simulink model "Longitudinaldynamicmodel_SmartFortwo"  (R2021b)
settings: Solver=FixedStepAuto  StartTime=0.0  StopTime=1  FixedStep=0.01  RelTol=1e-3
undefined symbols (not defined in the file): DiscIntNeverNeededParam, VehMass
libraries: Constant_Environment x1, Driver_PI x1, Longitudinal_DrivingCycles x1, Acceleration_Calculation x1, Air_Resistance x1, Roll_Resistance x1, Slope_Resistance x1, Constant_Power_Source x1, Simple_Auxiliary x1, Electric_Drive_Tabled_Consumption x1, Gear_Stage x1, DCAC_Converter x1
(part 2 of 3)

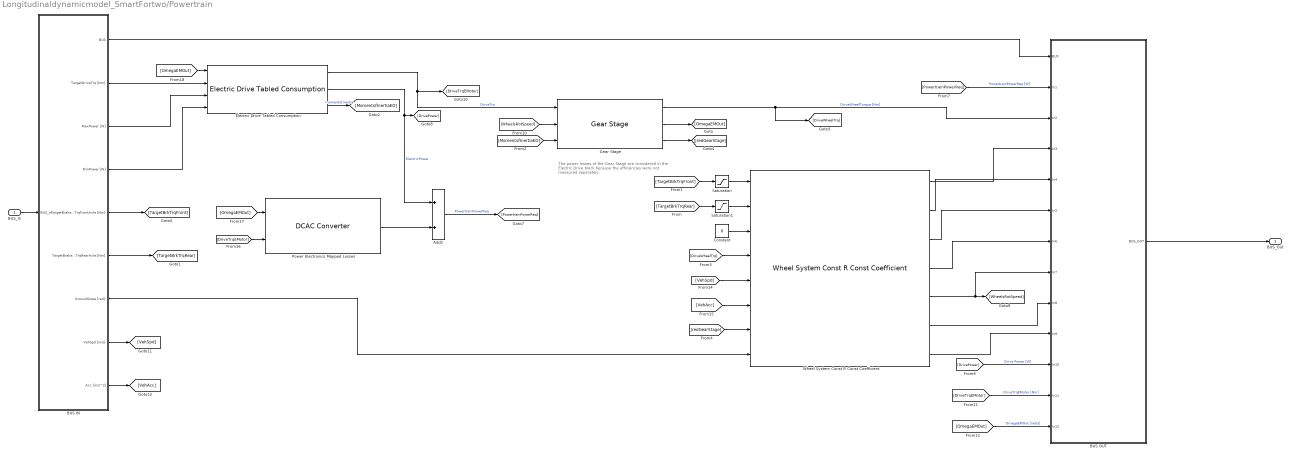
== system Longitudinaldynamicmodel_SmartFortwo/Powertrain ==
  note: The power losses of the Gear Stage are considered
      | in the Electric Drive block because the efficiencies were
      | not measured separately.
  BUS_In : Inport
  Add2 : Sum
  BUS IN : Subsystem
      mask help:
      | <Author> Alexander Koch based on Stefan Müller, Stephan Rohr
      | <Date> 02/05/2017
      |
      | <Description>
      | Automated BUS IN Block for the Bus System. After the Bus In is connected and receives signals it is possible to choose the required signals by clicking on the block. After choosing the signals it is possible to push the Refresh button. This button builds the required amount of outputs, connects the Bus Selector and the Outputs and rename all the outputs with the corresponding signal name.
      |
      | The Block automaticlly disconnects the link to the library block after opening the first time
      |
      | <Parameters>
      | -
      |
      | <Inputs>
      | Bus [Bus]
      |
      | <Outputs>
      | Bus [Bus]
      | SignalName[-]
      mask init:
      | BusInInitFct()
      settings: OpenFcn=|
      | set_param(gcb(),'LinkStatus','none')
      | open_system(gcb(),'mask')
      | open_system(strcat(gcb(),'/Bus Selector'),'Parameter')
      mask DialogControl ParameterGroupVar Prompt: Refresh
      mask DialogControl RefreshOutputs Prompt: Refresh all Output Names
      mask DialogControl RefreshOutputs Callback: BusInInitFct()
  BUS OUT : Subsystem  mask{NumberofInputs=12, NameSys='Powertrain'}
      mask prompts: NumberofInputs "Numper of costum inputs"; NameSys "Name of Bus Subsystem"
      mask help:
      | <Author> Alexander Koch based on Stefan Müller, Stephan Rohr
      | <Date> 02/05/2017
      |
      | <Description>
      | Automated BUS Out Block for the Bus System. Allows to enter the Number of costum inputs and the name of the bus system. After entering the parameters the required amout of Inputs are built and connected to the Bus Creator. The signal names that are connected to the inputs In1, ..., InN are automatically adopted at the Bus signal names and can be found in the Bus under the name of the Bus Subsystem. If the signal (line) to the Inport has no name, the name of the previous blocks outport is taken. If this is not possible, the name if the previous block is taken for the Bus signal name.
      |
      | Additional, there are two buttons. The Refresh Input Names refreshes all Input Names. This is required if signal names are changed or signals are connected for the first time. To build a new system or if another Subsystem is added between existing subsystems, the Refresh Bus Selector is required at every subsystem that is calculated after the new subsystem.
      |
      | The Block automaticlly disconnects the link to the library block after opening the first time
      |
      | <Parameters>
      | Number of costum inputs [-]
      | Name of Bus Subsystem ['abc']
      |
      | <Inputs>
      | Bus [Bus]
      | In1 [ ]
      |
      | <Outputs>
      | Bus [Bus]
      mask init:
      | BusRefreshInputs()
      settings: OpenFcn=|
      | set_param(gcb(),'LinkStatus','none')
      | open_system(gcb(),'mask')
      mask DialogControl Container3 Prompt: Refresh
      mask DialogControl RefreshInputNames Prompt: Refresh Input Names
      mask DialogControl RefreshInputNames Callback: BusRefreshLineNames()
      mask DialogControl RefreshBusSelector Prompt: Refresh Bus Selector
      mask DialogControl RefreshBusSelector Callback: BusRefreshBusSelector()
  Constant : Constant  Value=0
  Electric Drive Tabled Consumption : Electric_Drive_Tabled_Consumption/Electric Drive Tabled Consumption  inertia=0.03  mass=1  OM_M_Pel_Map=[-4936.58960230285,-4918.30593710914,-4900.02227191542,-4881.73860672171,-4863.45494152799,-4845.17127633428,-4826.88761114056,-4808.60394594685,-4790.32028075314,-4772.03661555942,-4753.75295036571,-4735.46928517199,-4717.18561997828,-4698.90195478456,-4680.61828959085,-4662.33462439714,-5185.11366506308,-5115.90505550168,-4971.88831379428,-4292.42207149109,-4491.53844424213,-4496.68242435772,-3427.33324656741,-3576.85553346338,-4862.92900152083,-6633.71124555647,-8634.89642494398,-4640.86226177616,-3090.77270566202,-3263.80065362687,-3496.71961565219,-3476.52721907770,-3156.42090156138,-3528.67393415159,-3943.07312633913,-1726.22025060580,0,-284.730200184838,-3008.08986597435,-2771.67771496470,-1854.05476499352,-1637.18751237163,-1896.50054154000,-1755.41745851923,-1704.42214651483,-1837.80488310502,-2503.90899285254,-3057.39048489453,-3952.42911160673,-4269.34747269463,-4242.89467363708,-4204.95309118347,-4162.48827607546,-4121.62290347057,-4107.04807601649,-4077.92876166182,-4033.68022948992,-4001.70150845442,-3928.04097239828,-3892.85157240146,-3860.86018153553,-3833.69713173239,-3822.33875240511,-3752.79975327265,-3710.92826749583,-3673.11813401635,-3650.11543119095,-3617.55425584301,-3571.83464080449,-3546.22881032664,-3521.91492991431,-3503.51647273559,-3486.02852972273,-3456.08511172243,-3426.20785526970,-3393.22836186158,-3347.26416827824,-3315.74459108047,-3296.14668080983,-3259.87537919135,-3239.41741836494,-3209.57517612393,-3171.72598576032,-3145.46589033245,-3114.73817397058,-3096.82260491367,-3083.69891203201,-3028.53546438293,-2988.91641709166,-2952.55258487163,-2929.27984242158,-2918.30740683215,-2873.01765728202,-2827.29316803929,-2793.78872353345,-2774.19345844693,-2759.15266733751,-2740.21288555482,-2712.48373689461,-2700.63324424749,-2672.00671871173,-2652.70867089400,-2641.22885174613,-2609.92742749761,-2590.43803114605,-2552.66583691581,-2523.45685997718,-2500.24253764220,-2459.00798676327,-2438.92186521623,-2407.06238415750,-2382.52048698444,-2363.76081048896,-2359.58944186339,-2345.68370297819,-2308.79818370909,-2284.46288528949,-2265.18882858931,-2236.12233498368,-2202.96158268492,-2190.88870254505,-2161.55169347863,-2130.75207473189,-2100.15228890542,-2083.00628884149,-2065.03289270050,-2037.48564486677,-2023.21148849436,-2003.60224940543,-1985.10896747608,-1973.43738121688,-1954.15563352281,-1936.49980013294,-1927.41778977736,-1881.51131814734,-1833.22793591959,-1812.31297236205,-1791.45842660955,-1776.91834015446,-1771.92258671922,-1753.46238532805,-1738.43989396041,-1734.97839912883,-1730.47565907493,-1707.15901890688,-1688.09192045326,-1670.78344209104,-1655.54467412356,-1639.03791207785,-1627.05930580792,-1604.77335708724,-1587.38076614672,-1561.52550139142,-1537.72571637804,-1510.39275514847,-1470.58244002962,-1453.15319676168,-1410.88893113516,-1321.00360833135,-1269.23703081773,-1254.49077239222,-1241.38468901509,-1229.32636706052,-1202.25203822531,-1184.94448226145,-1158.42848336410,-1136.20405147524,-1126.39720329839,-1106.37247296839,-1094.85258153359,-1077.77222327341,-1048.86179199116,-1029.92385889766,-1012.51433236396,-1002.83703023995,-999.671500372368,-987.625469219025,-971.502457237745,-944.816892286739,-933.727512080550,-927.465392779959,-908.500787820009,-892.918090905503,-877.260552760021,-857.206260698465,-846.212481472991,-838.179969253041,-830.641165096547,-807.984200911199,-798.124054496656,-792.518428146118,-765.637990495186,-746.212652936259,-712.453130410888,-696.980692898239,-691.969161426306,-672.764183049685,-663.434558579034,-643.975843820281,-631.350187559368,-617.856740921016,-610.270426732149,-591.410647728663,-578.788040954300,-569.720295539698,-556.273882509573,-549.087372350833,-540.864224298053,-525.831584341530,-513.205249528202,-497.309584323254,-484.661307411820,-466.385751839651,-461.707756868834,-448.056335365480,-434.987633724325,-427.031177729718,-408.480763130817,-385.296760841008,-359.496386063347,-344.092316830198,-331.596273553197,-323.279256624167 ...(+563781 chars)]  M_MotVector=[-135,-134.500000000000,-134,-133.500000000000,-133,-132.500000000000,-132,-131.500000000000,-131,-130.500000000000,-130,-129.500000000000,-129,-128.500000000000,-128,-127.500000000000,-127,-126.500000000000,-126,-125.500000000000,-125,-124.500000000000,-124,-123.500000000000,-123,-122.500000000000,-122,-121.500000000000,-121,-120.500000000000,-120,-119.500000000000,-119,-118.500000000000,-118,-117.500000000000,-117,-116.500000000000,-116,-115.500000000000,-115,-114.500000000000,-114,-113.500000000000,-113,-112.500000000000,-112,-111.500000000000,-111,-110.500000000000,-110,-109.500000000000,-109,-108.500000000000,-108,-107.500000000000,-107,-106.500000000000,-106,-105.500000000000,-105,-104.500000000000,-104,-103.500000000000,-103,-102.500000000000,-102,-101.500000000000,-101,-100.500000000000,-100,-99.5000000000000,-99,-98.5000000000000,-98,-97.5000000000000,-97,-96.5000000000000,-96,-95.5000000000000,-95,-94.5000000000000,-94,-93.5000000000000,-93,-92.5000000000000,-92,-91.5000000000000,-91,-90.5000000000000,-90,-89.5000000000000,-89,-88.5000000000000,-88,-87.5000000000000,-87,-86.5000000000000,-86,-85.5000000000000,-85,-84.5000000000000,-84,-83.5000000000000,-83,-82.5000000000000,-82,-81.5000000000000,-81,-80.5000000000000,-80,-79.5000000000000,-79,-78.5000000000000,-78,-77.5000000000000,-77,-76.5000000000000,-76,-75.5000000000000,-75,-74.5000000000000,-74,-73.5000000000000,-73,-72.5000000000000,-72,-71.5000000000000,-71,-70.5000000000000,-70,-69.5000000000000,-69,-68.5000000000000,-68,-67.5000000000000,-67,-66.5000000000000,-66,-65.5000000000000,-65,-64.5000000000000,-64,-63.5000000000000,-63,-62.5000000000000,-62,-61.5000000000000,-61,-60.5000000000000,-60,-59.5000000000000,-59,-58.5000000000000,-58,-57.5000000000000,-57,-56.5000000000000,-56,-55.5000000000000,-55,-54.5000000000000,-54,-53.5000000000000,-53,-52.5000000000000,-52,-51.5000000000000,-51,-50.5000000000000,-50,-49.5000000000000,-49,-48.5000000000000,-48,-47.5000000000000,-47,-46.5000000000000,-46,-45.5000000000000,-45,-44.5000000000000,-44,-43.5000000000000,-43,-42.5000000000000,-42,-41.5000000000000,-41,-40.5000000000000,-40,-39.5000000000000,-39,-38.5000000000000,-38,-37.5000000000000,-37,-36.5000000000000,-36,-35.5000000000000,-35,-34.5000000000000,-34,-33.5000000000000,-33,-32.5000000000000,-32,-31.5000000000000,-31,-30.5000000000000,-30,-29.5000000000000,-29,-28.5000000000000,-28,-27.5000000000000,-27,-26.5000000000000,-26,-25.5000000000000,-25,-24.5000000000000,-24,-23.5000000000000,-23,-22.5000000000000,-22,-21.5000000000000,-21,-20.5000000000000,-20,-19.5000000000000,-19,-18.5000000000000,-18,-17.5000000000000,-17,-16.5000000000000,-16,-15.5000000000000,-15,-14.5000000000000,-14,-13.5000000000000,-13,-12.5000000000000,-12,-11.5000000000000,-11,-10.5000000000000,-10,-9.50000000000000,-9,-8.50000000000000,-8,-7.50000000000000,-7,-6.50000000000000,-6,-5.50000000000000,-5,-4.50000000000000,-4,-3.50000000000000,-3,-2.50000000000000,-2,-1.50000000000000,-1,-0.500000000000000,0,0.500000000000000,1,1.50000000000000,2,2.50000000000000,3,3.50000000000000,4,4.50000000000000,5,5.50000000000000,6,6.50000000000000,7,7.50000000000000,8,8.50000000000000,9,9.50000000000000,10,10.5000000000000,11,11.5000000000000,12,12.5000000000000,13,13.5000000000000,14,14.5000000000000,15,15.5000000000000,16,16.5000000000000,17,17.5000000000000,18,18.5000000000000,19,19.5000000000000,20,20.5000000000000,21,21.5000000000000,22,22.5000000000000,23,23.5000000000000,24,24.5000000000000,25,25.5000000000000,26,26.5000000000000,27,27.5000000000000,28,28.5000000000000,29,29.5000000000000,30,30.5000000000000,31,31.5000000000000,32,32.5000000000000,33,33.5000000000000,34,34.5000000000000,35,35.5000000000000,36,36.5000000000000,37,37.5000000000000,38,38.5000000000000,39,39.5000000000000,40,40.5000000000000,41,41.5000000000000,42,42.5000000000000,43,43.5000000000000,44,44.5000000000000,45,45.5000000000000,46,46.5000000000000,47,47.5000000000000,48,48.5000000000000,49,49.5000000000000,50 ...(+1736 chars)]  OM_MotVector=[0,11.6256677293860,23.2513354587719,34.8770031881579,46.5026709175438,58.1283386469298,69.7540063763158,81.3796741057017,93.0053418350877,104.631009564474,116.256677293860,127.882345023246,139.508012752632,151.133680482017,162.759348211403,174.385015940789,186.010683670175,197.636351399561,209.262019128947,220.887686858333,232.513354587719,244.139022317105,255.764690046491,267.390357775877,279.016025505263,290.641693234649,302.267360964035,313.893028693421,325.518696422807,337.144364152193,348.770031881579,360.395699610965,372.021367340351,383.647035069737,395.272702799123,406.898370528509,418.524038257894,430.149705987280,441.775373716666,453.401041446052,465.026709175438,476.652376904824,488.278044634210,499.903712363596,511.529380092982,523.155047822368,534.780715551754,546.406383281140,558.032051010526,569.657718739912,581.283386469298,592.909054198684,604.534721928070,616.160389657456,627.786057386842,639.411725116228,651.037392845614,662.663060575000,674.288728304386,685.914396033772]  M_Full_Load=[128 128 128 127 127 126 126 126 126 124 119 114 109 103 100 94 89 85 79 75 70 68 67 65 63 62 60 58 59 60 62 63 63 62 61 60 58 57 55 53 51 50 48 46 45 43 42 40 39 38 36 35 34 32 31 30 29 28 26 25 24]  OM_Full_Load=[0 11.4144533080429 22.8289066160858 34.2433599241288 45.6578132321717 57.1769862953342 68.5914396033771 80.0058929114201 91.4203462194630 102.834799527506 114.249252835549 125.663706143592 137.078159451635 148.492612759678 160.011785822840 171.426239130883 182.840692438926 194.255145746969 205.669599055012 217.084052363055 228.498505671098 239.912958979141 251.327412287183 262.846585350346 274.261038658389 285.675491966432 297.089945274475 308.504398582518 319.918851890561 331.333305198604 342.747758506646 354.162211814689 365.681384877852 377.095838185895 388.510291493938 399.924744801981 411.339198110024 422.753651418066 434.168104726109 445.582558034152 456.997011342195 468.516184405358 479.930637713401 491.345091021444 502.759544329487 514.173997637529 525.588450945572 537.002904253615 548.417357561658 559.831810869701 571.350983932864 582.765437240907 594.179890548950 605.594343856992 617.008797165035 628.423250473078 639.837703781121 651.252157089164 662.666610397207 674.185783460370 685.600236768413]  M_Min_Load=[0 0 0 0 0 0 0 0 0 0 0 0 0 0 0 0 0 0 0 0 0 0 0 0 0 0 0 0 0 0 0 0 0 0 0 0 0 0 0 0 0 0 0 0 0 0 0 0 0 0 0 0 0 0 0 0 0 0 0 0 0]  OM_Min_Load=[0 11.4144533080429 22.8289066160858 34.2433599241288 45.6578132321717 57.1769862953342 68.5914396033771 80.0058929114201 91.4203462194630 102.834799527506 114.249252835549 125.663706143592 137.078159451635 148.492612759678 160.011785822840 171.426239130883 182.840692438926 194.255145746969 205.669599055012 217.084052363055 228.498505671098 239.912958979141 251.327412287183 262.846585350346 274.261038658389 285.675491966432 297.089945274475 308.504398582518 319.918851890561 331.333305198604 342.747758506646 354.162211814689 365.681384877852 377.095838185895 388.510291493938 399.924744801981 411.339198110024 422.753651418066 434.168104726109 445.582558034152 456.997011342195 468.516184405358 479.930637713401 491.345091021444 502.759544329487 514.173997637529 525.588450945572 537.002904253615 548.417357561658 559.831810869701 571.350983932864 582.765437240907 594.179890548950 605.594343856992 617.008797165035 628.423250473078 639.837703781121 651.252157089164 662.666610397207 674.185783460370 685.600236768413]  LocalSampleTime=-1
  Gear Stage : Gear_Stage/Gear Stage  iGear=i_gear  eta=1  JredGetr=0.19  LocalSampleTime=-1
  Power Electronics Mapped Losses : DCAC_Converter/DCAC Converter  W_Vektor=[0 10.4719755119660 21.7817090648892 33.0914426178125 44.4011761707357 55.7109097236590 67.0206432765823 78.3303768295055 89.6401103824288 100.949843935352 112.259577488275 123.569311041199 134.879044594122 146.188778147045 157.498511699968 168.808245252892 180.117978805815 191.427712358738 202.737445911661 214.047179464585 225.356913017508 236.666646570431 247.976380123354 259.286113676278 270.595847229201 281.905580782124 293.215314335047 304.525047887971 315.834781440894 327.144514993817 338.454248546740 349.763982099664 361.073715652587 372.383449205510 383.693182758433 395.002916311357 406.312649864280 417.622383417203 428.932116970126 440.241850523050 451.551584075973 462.861317628896 474.171051181819 485.480784734743 496.790518287666 508.100251840589 519.409985393512 530.719718946436 542.029452499359 553.339186052282 564.648919605206 575.958653158129 587.268386711052 598.578120263975 609.887853816898 621.197587369822 632.507320922745 643.817054475668 655.126788028592 666.436521581515 677.746255134438]  M_Vektor_motgen=[0 1 2 3 4 5 6 7 8 9 10 11 12 13 14 15 16 17 18 19 20 21 22 23 24 25 26 27 28 29 30 31 32 33 34 35 36 37 38 39 40 41 42 43 44 45 46 47 48 49 50 51 52 53 54 55 56 57 58 59 60 61 62 63 64 65 66 67 68 69 70 71 72 73 74 75 76 77 78 79 80 81 82 83 84 85 86 87 88 89 90 91 92 93 94 95 96 97 98 99 100 101 102 103 104 105 106 107 108 109 110 111 112 113 114 115 116 117 118 119 120 121 122 123 124 125 126 127 128 129 130]  P_Loss=[0 0 0 0 0 0 0 0 0 0 0 0 0 0 0 0 0 0 0 0 0 0 0 0 0 0 0 0 0 0 0 0 0 0 0 0 0 0 0 0 0 0 0 0 0 0 0 0 0 0 0 0 0 0 0 0 0 0 0 0 0 0 0 0 0 0 0 0 0 0 0 0 0 0 0 0 0 0 0 0 0 0 0 0 0 0 0 0 0 0 0 0 0 0 0 0 0 0 0 0 0 0 0 0 0 0 0 0 0 0 0 0 0 0 0 0 0 0 0 0 0 0 0 0 0 0 0 0 0 0 0;0 82 70 84 90 100 106 112 101 115 122 130 144 146 153 162 154 169 188 198 202 216 231 236 247 260 271 279 293 309 316 326 335 353 373 392 407 427 437 460 475 478 493 505 523 529 551 565 570 582 598 616 631 647 665 682 700 716 730 726 743 763 780 805 824 840 861 884 903 919 947 960 981 995 1018 1041 1062 1086 1110 1130 1152 1170 1188 1211 1237 1259 1280 1302 1323 1344 1369 1392 1412 1440 1460 1493 1518 1540 1568 1594 1617 1646 1670 1709 1743 1769 1791 1825 1856 1881 1938 2212 3001 3444 3441 3510 3626 3825 3876 3879 3957 4140 4177 3954 4094 3971 3839 3839 3839 3839 3839;0 61 78 75 74 73 81 94 94 97 96 106 120 131 139 145 154 169 180 188 198 206 215 230 242 254 265 268 286 302 306 318 344 370 384 399 410 423 438 458 483 500 512 520 528 539 554 573 589 600 614 632 645 655 678 691 714 720 739 748 763 777 787 809 833 829 860 887 913 937 949 962 976 988 1007 1032 1049 1076 1095 1118 1143 1168 1192 1212 1231 1256 1293 1323 1337 1356 1387 1406 1427 1456 1469 1496 1515 1558 1577 1607 1643 1675 1694 1710 1739 1772 1805 1832 1870 1893 1924 1942 1976 1999 2049 2640 3767 4034 4108 4084 4241 4351 4407 4486 4544 4620 3839 3839 3839 3839 3839;0 70 71 95 83 94 92 96 105 107 112 125 141 143 150 153 165 176 190 203 218 233 240 245 253 260 274 285 304 329 341 352 358 365 379 403 424 444 460 472 483 499 525 535 543 561 575 589 597 611 632 643 656 664 677 700 719 731 742 759 777 794 814 839 858 870 892 917 938 953 968 987 1008 1022 1035 1055 1085 1111 1129 1151 1176 1192 1213 1240 1276 1296 1325 1348 1369 1387 1405 1432 1465 1493 1507 1525 1558 1586 1614 1642 1663 1683 1718 1753 1777 1801 1832 1860 1893 1925 1956 1984 2007 2030 2062 2093 2124 2160 2187 2222 2252 2304 2714 4353 4916 3997 3839 3839 3839 3839 3839;0 74 50 130 190 192 101 114 128 71 125 147 164 97 157 185 186 201 216 227 232 238 241 252 264 279 293 306 320 335 355 350 365 394 396 405 423 436 452 468 481 497 508 518 532 545 554 569 588 604 613 625 645 667 677 690 709 726 745 765 780 791 803 829 843 855 881 897 912 926 942 967 994 1017 1036 1056 1073 1104 1121 1152 1181 1210 1240 1264 1282 1303 1323 1349 1371 1396 1415 1439 1469 1495 1515 1540 1563 1591 1625 1648 1677 1706 1736 1764 1793 1824 1842 1877 1912 1945 1975 2002 2024 2048 2081 2116 2143 2180 2207 2259 2278 2340 2348 2402 2412 3130 3839 3839 3839 3839 3839;0 97 63 80 77 71 70 92 102 101 123 143 135 155 167 123 148 166 185 200 226 242 265 255 265 280 315 323 318 335 346 366 381 399 417 422 439 455 469 485 498 512 525 539 550 574 587 589 608 620 642 662 668 685 705 718 725 738 758 776 792 805 834 852 859 885 897 923 947 967 985 998 1012 1023 1052 1079 1100 1125 1143 1167 1187 1214 1253 1276 1309 1333 1360 1375 1400 1424 1445 1464 1482 1504 1536 1562 1591 1615 1648 1680 1708 1734 1763 1796 1819 1825 1852 1870 1910 1946 1979 2013 2048 2088 2118 2153 2189 2216 2239 2276 2311 2337 2377 2430 2439 3130 3839 3839 3839 3839 3839;0 54 47 58 68 60 51 67 76 84 98 114 113 116 128 138 140 157 175 171 180 195 214 221 231 239 258 265 274 290 315 334 355 377 405 415 432 449 467 482 502 518 521 532 552 558 572 584 600 622 634 651 666 679 694 714 726 740 762 782 800 820 833 853 876 894 914 931 953 971 981 991 1011 1036 1068 1088 1111 1128 1142 1166 1197 1229 1255 1273 1304 1348 1379 1414 1440 1454 1475 1496 1514 1537 1564 1589 1611 1605 1652 1678 1706 1735 1768 1805 1835 1862 1903 1936 1962 2002 2036 2057 2079 2113 2149 2183 2212 2244 2285 2323 2355 2386 2410 2437 2457 3130 3839 3839 3839 3839 3839;0 78 78 96 96 93 93 106 115 120 127 134 146 157 157 161 179 196 182 188 211 212 224 245 260 287 306 309 317 325 338 356 376 399 405 416 447 470 487 494 492 494 517 534 542 561 575 584 604 625 635 656 668 681 703 723 742 765 786 804 816 829 843 864 889 904 916 929 942 962 992 1019 1036 1061 1082 ...(+31348 chars)]  LocalSampleTime=-1
  Saturation : Saturate  UpperLimit=0  LowerLimit=-inf
  Saturation1 : Saturate  UpperLimit=0  LowerLimit=-inf
  Wheel System Const R Const Coefficient : Wheel_System_Const_R/Wheel System Const R Const Coefficient  Wheel_Radius=r_dyn  Wheel_Roll_Resistance=0.0185  Wheel_Roll_Resistance_Dyn=0  mu_Tyre=0.7  J_FourWheels=4  Gravity=gravity  Wheelbase=1.863  COG_Height=0.5  COG_Front=1.1178  COG_Rear=0.7452  Veh_Mass=VehMass  LocalSampleTime=-1
  BUS_Out : Outport  VectorParamsAs1DForOutWhenUnconnected=off
  wires:
  BUS IN/1(BUS) -> BUS OUT/1(BUS)
  BUS_In/1 -> BUS IN/1(BUS_In)
  [TargetBrkTrqFront] -> Saturation/1
  [TargetBrkTrqRear] -> Saturation1/1
  BUS IN/5(TargetBrakeTrqFrontAxle [Nm]) -> [TargetBrkTrqFront]
  BUS IN/2(TargetDriveTrq [Nm]) -> Electric Drive Tabled Consumption/2
  Electric Drive Tabled Consumption/1 -> Gear Stage/1, [DriveTrqEMotor]  "DriveTrq"
  Gear Stage/2 -> [OmegaEMOut]
  Constant/1 -> Wheel System Const R Const Coefficient/3
  [MomentofInertiaED] -> Gear Stage/3
  Gear Stage/1 -> [DriveWheelTrq], BUS OUT/3(In2)  "DriveWheelTorque [Nm]"
  [DriveWheelTrq] -> Wheel System Const R Const Coefficient/4
  Gear Stage/3 -> [JredGearStage]
  [JredGearStage] -> Wheel System Const R Const Coefficient/7
  Wheel System Const R Const Coefficient/1 -> BUS OUT/4(In3)
  Wheel System Const R Const Coefficient/2 -> BUS OUT/5(In4)
  Wheel System Const R Const Coefficient/3 -> BUS OUT/6(In5)
  Wheel System Const R Const Coefficient/4 -> BUS OUT/7(In6)
  Wheel System Const R Const Coefficient/5 -> [WheelsRotSpeed], BUS OUT/8(In7)
  Wheel System Const R Const Coefficient/6 -> BUS OUT/9(In8)
  Wheel System Const R Const Coefficient/7 -> BUS OUT/10(In9)
  Electric Drive Tabled Consumption/2 -> Add2/1, [DrivePower]  "ElectricPower"
  Add2/1 -> [PowertrainPowerReq]  "PowertrainPowerReq"
  BUS IN/7(GroundSlope [rad]) -> Wheel System Const R Const Coefficient/8
  Saturation/1 -> Wheel System Const R Const Coefficient/1
  Saturation1/1 -> Wheel System Const R Const Coefficient/2
  [PowertrainPowerReq] -> BUS OUT/2(In1)  "PowertrainPowerReq [W]"
  [DrivePower] -> BUS OUT/11(In10)  "Drive Power [W]"
  [WheelsRotSpeed] -> Gear Stage/2
  [DriveTrqEMotor] -> BUS OUT/12(In11)  "DriveTrqEMotor [Nm]"
  [OmegaEMOut] -> BUS OUT/13(In12)  "OmegaEMOut [rad/s]"
  BUS IN/6(TargetBrakeTrqRearAxle [Nm]) -> [TargetBrkTrqRear]
  BUS IN/8(VehSpd [m/s]) -> [VehSpd]
  [VehSpd] -> Wheel System Const R Const Coefficient/5
  BUS IN/9(Acc [m/s^2]) -> [VehAcc]
  [VehAcc] -> Wheel System Const R Const Coefficient/6
  [DriveTrqEMotor] -> Power Electronics Mapped Losses/2
  [OmegaEMOut] -> Power Electronics Mapped Losses/1
  Power Electronics Mapped Losses/1 -> Add2/2
  [OmegaEMOut] -> Electric Drive Tabled Consumption/1
  Electric Drive Tabled Consumption/3 -> [MomentofInertiaED]  "momentofinertia"
  BUS IN/3(MaxPower [W]) -> Electric Drive Tabled Consumption/3
  BUS IN/4(MinPower [W]) -> Electric Drive Tabled Consumption/4
  BUS OUT/1(BUS_OUT) -> BUS_Out/1
